simulink model "siWDqudong_FAN_MPC"  (R2024b)
settings: Solver=ode4  StartTime=0.0  StopTime=30  FixedStep=0.0005  RelTol=1e-3
undefined symbols (not defined in the file): MotorData, Q_beta_tune, Q_yaw_tune, R_alloc_tune, R_rate_tune, Road_Curvature_Map, Road_Mu_Map, Sim_Mu_Set, Sim_Vx_Set, Target_Speed_Map, W_util_tune
libraries: Solver_SF x1
(part 3 of 3)

== matlab function siWDqudong_FAN_MPC/Subsystem1/MATLAB Function ==
  data: x_curr input; T_final_opt output; Solver_Status output; x_ref input; T_ref_upper_in input size=[4 1]; Vehicle_State input; Stiffness_Input input size=[2 1]; NN_Weights input; Constraints input; dt_in input; Mu_in input; Curv_in input; Delta_f_in input; Debug_Info output size=[5 1]
function [T_final_opt, Solver_Status, Debug_Info] = Lower_Layer_MPC_Fixed(...
    x_curr, x_ref, T_ref_upper_in, Vehicle_State, Stiffness_Input, ...
    NN_Weights, Constraints, dt_in, Mu_in, Curv_in, Delta_f_in)
%#codegen
% =========================================================================
% 下层四轮LTV-MPC V6.2 dynamic W_util
%
% 直接替换原 Lower_Layer_MPC_Fixed。
% 输入/输出接口保持不变。
%
% 主要修正：
% 1) 使用可解释的无量纲物理归一化cost；
% 2) Np=25, Nc=2，Nc以后保持最后控制量；
% 3) 真正硬约束：
%       |u1-u_prev| <= dT_rate_max*dt
%       |u2-u1|     <= dT_rate_max*dt
% 4) Constraints(3) 明确定义为 Nm/s。
%    若 Constraints=[-200,800,600] 且dt=0.01，则du_max=6 Nm/step；
% 5) 不再使用8000 Nm/s的默认超大变化率去“放任抖振”；
% 6) 电机上下限使用Constraints(1/2)，同时仍限制到车辆实际±350 Nm范围；
% 7) BO/BPNN权重为无量纲乘子；搜索域与V5归一化定义同步；
% 8) fallback优先满足当前轮胎/电机安全边界；
% 9) 参考转矩只做轻度低通，避免与上层形成过重双重延迟。
% 10) 原 W_slip 重构为 W_util：按每轮动态剩余纵向能力连续归一化，无固定软阈值。
% =========================================================================

%% 0. 初始化
T_final_opt = zeros(4,1,'double');
Solver_Status = 0.0;
Debug_Info = zeros(5,1,'double');

%% 1. 输入
Veh_State = double(reshape(Vehicle_State,6,1));

Vx = max(Veh_State(1),1.0);

Fz_floor = 100.0;
Fz_fl_raw = max(Veh_State(3),Fz_floor);
Fz_fr_raw = max(Veh_State(4),Fz_floor);
Fz_rl_raw = max(Veh_State(5),Fz_floor);
Fz_rr_raw = max(Veh_State(6),Fz_floor);

dt = double(dt_in(1));
if dt <= 0
    dt = 0.01;
end

beta_in = double(x_curr(1));
r_in = double(x_curr(2));
x_ref_safe = double(reshape(x_ref,2,1));

delta_f_rad = double(Delta_f_in(1));

mu_est = min(max(double(Mu_in(1)),0.15),1.20);

kappa_abs = abs(double(Curv_in(1)));

%% 2. persistent
persistent u_prev
persistent Fz_fl_f Fz_fr_f Fz_rl_f Fz_rr_f
persistent T_ref_f
persistent logW_prev
persistent weight_initialized

if isempty(u_prev)
    u_prev = zeros(4,1);

    Fz_fl_f = Fz_fl_raw;
    Fz_fr_f = Fz_fr_raw;
    Fz_rl_f = Fz_rl_raw;
    Fz_rr_f = Fz_rr_raw;

    T_ref_f = double(reshape(T_ref_upper_in,4,1));

    logW_prev = [log10(2000.0);log10(125.0);log10(3000.0);log10(480.0);log10(1.0)];
    weight_initialized = false;
end

%% 3. Fz滤波
tau_Fz = 0.06;
alpha_Fz = dt/(tau_Fz+dt);

Fz_fl_f = Fz_fl_f + alpha_Fz*(Fz_fl_raw-Fz_fl_f);
Fz_fr_f = Fz_fr_f + alpha_Fz*(Fz_fr_raw-Fz_fr_f);
Fz_rl_f = Fz_rl_f + alpha_Fz*(Fz_rl_raw-Fz_rl_f);
Fz_rr_f = Fz_rr_f + alpha_Fz*(Fz_rr_raw-Fz_rr_f);

Fz_fl = Fz_fl_f;
Fz_fr = Fz_fr_f;
Fz_rl = Fz_rl_f;
Fz_rr = Fz_rr_f;

Fz_total = Fz_fl+Fz_fr+Fz_rl+Fz_rr;

% 硬安全边界使用raw和filtered中较保守者
Fz_fl_safe = max(min(Fz_fl_raw,Fz_fl_f),Fz_floor);
Fz_fr_safe = max(min(Fz_fr_raw,Fz_fr_f),Fz_floor);
Fz_rl_safe = max(min(Fz_rl_raw,Fz_rl_f),Fz_floor);
Fz_rr_safe = max(min(Fz_rr_raw,Fz_rr_f),Fz_floor);

%% 4. 上层参考只做轻度平滑
T_ref_raw = double(reshape(T_ref_upper_in,4,1));

tau_ref = 0.035;
alpha_ref = dt/(tau_ref+dt);

T_ref_f = T_ref_f + alpha_ref*(T_ref_raw-T_ref_f);

T_ref_upper = T_ref_f;
T_total_req = sum(T_ref_upper);

%% 5. 权重：BO训练域投影 + log变化率限制
W_in = double(reshape(NN_Weights,5,1));
W_in = max(W_in,1e-12);

logW_raw = log10(W_in);

log_lo = [0.0;0.7958800173;1.0;-3.0;-3.0];
log_hi = [4.5;3.2958800173;5.5;3.7041199827;4.0];

for ii=1:5
    logW_raw(ii)=min(max(logW_raw(ii),log_lo(ii)),log_hi(ii));
end

dlog_max = [0.08;0.08;0.10;0.10;0.10];

if ~weight_initialized
    logW_eff = logW_raw;
    weight_initialized = true;
else
    dlog = logW_raw-logW_prev;

    for ii=1:5
        dlog(ii)=min(max(dlog(ii),-dlog_max(ii)),dlog_max(ii));
    end

    logW_eff = logW_prev+dlog;
end

logW_prev = logW_eff;

W_eff = 10.^logW_eff;

Q_beta_raw  = W_eff(1);
Q_yaw_raw   = W_eff(2);
R_alloc_raw = W_eff(3);
R_rate_raw  = W_eff(4);
W_util_raw  = W_eff(5);

%% 6. 物理归一化
% Characteristic scales for dimensionless MPC cost
% beta_s : characteristic sideslip error [rad]
% r_s    : characteristic yaw-rate tracking error [rad/s]
% T_s    : characteristic single-wheel torque error [Nm]
% dT_s   : nominal one-step torque increment at 2000 Nm/s, dt=0.01 s [Nm]
% Tsum_s : four-wheel total-torque characteristic scale [Nm]
beta_s = 0.05;
r_s    = 0.10;
T_s    = 100.0;
dT_s   = 20.0;
Tsum_s = 400.0;

Q_beta = Q_beta_raw/(beta_s^2);
Q_yaw  = Q_yaw_raw /(r_s^2);

R_alloc = R_alloc_raw/(T_s^2);

R_rate_base = R_rate_raw/(dT_s^2);
R_rate_vec = R_rate_base*ones(4,1);

% q_sum is rescaled from the old 90000/320^2 so the working baseline
% effective total-demand penalty is exactly preserved after Tsum_s=400 Nm.
W_sum = 140625.0/(Tsum_s^2);

Re = 0.347;

% V6.2: dynamic remaining longitudinal tire capacity.
% No fixed 0.80/0.85 utilization threshold is used. The soft penalty grows
% continuously as mu decreases, Fz unloads, or lateral demand increases.
D_lat = Vx*Vx*kappa_abs/max(mu_est*9.81,1e-6);
gamma_mu = 1.00;  % physical friction-circle boundary, not a soft threshold
friction_factor = sqrt(max(gamma_mu^2-D_lat^2,0.0));

T_dyn_fl = Fz_fl_safe*mu_est*friction_factor*Re;
T_dyn_fr = Fz_fr_safe*mu_est*friction_factor*Re;
T_dyn_rl = Fz_rl_safe*mu_est*friction_factor*Re;
T_dyn_rr = Fz_rr_safe*mu_est*friction_factor*Re;

% Smooth denominator prevents numerical singularity without introducing a
% fixed switching threshold. J_util ~= W_util * sum((T_i/T_cap_i)^2).
T_util_eps = 5.0;
T_util_scale = sqrt([T_dyn_fl^2;T_dyn_fr^2;T_dyn_rl^2;T_dyn_rr^2] + T_util_eps^2);
W_util_vec = W_util_raw./(T_util_scale.^2);

%% 7. LTV模型
Cf = max(double(Stiffness_Input(1)),1000.0);
Cr = max(double(Stiffness_Input(2)),1000.0);

Np = 25;
Nc = 2;
nx = 2;
nu = 4;

m  = 1810.0;
Iz = 2765.0;
lf = 1.152;
lr = 1.528;
twf = 1.565;
twr = 1.565;

a11 = -(Cf+Cr)/(m*Vx);
a12 = ((lr*Cr-lf*Cf)/(m*Vx^2))-1.0;
a21 = (lr*Cr-lf*Cf)/Iz;
a22 = -(lf^2*Cf+lr^2*Cr)/(Iz*Vx);

A = eye(nx)+[a11,a12;a21,a22]*dt;

B_row2 = [ ...
    -twf/(2*Re*Iz), ...
     twf/(2*Re*Iz), ...
    -twr/(2*Re*Iz), ...
     twr/(2*Re*Iz)]*dt;

B = [zeros(1,4);B_row2];

B_delta_cont = [Cf/(m*Vx);lf*Cf/Iz];
B_delta = B_delta_cont*dt;

%% 8. 预测矩阵
Phi = zeros(nx*Np,nx);
Gamma = zeros(nx*Np,nu*Nc);
Gamma_delta = zeros(nx*Np,1);

for i=1:Np
    rows_i=(i-1)*nx+(1:nx);

    Phi(rows_i,:)=A^i;

    % steering在预测域中保持当前值
    Gd=zeros(nx,1);
    for q=0:(i-1)
        Gd=Gd+(A^q)*B_delta;
    end
    Gamma_delta(rows_i,:)=Gd;

    for j=1:min(i,Nc)
        cols_j=(j-1)*nu+(1:nu);

        if j < Nc
            term=(A^(i-j))*B;
        else
            % 第Nc个控制量保持至预测域结束
            term=zeros(nx,nu);

            for q=0:(i-Nc)
                term=term+(A^q)*B;
            end
        end

        Gamma(rows_i,cols_j)=term;
    end
end

%% 9. Cost
Q_bar = kron(eye(Np),diag([Q_beta;Q_yaw]));

H_stab = Gamma'*Q_bar*Gamma;

X_free = Phi*[beta_in;r_in]+Gamma_delta*delta_f_rad;
Y_ref = repmat(x_ref_safe,Np,1);

f_stab = (X_free-Y_ref)'*Q_bar*Gamma;

% 9.1 nominal torque reference
R_alloc_mat = diag(repmat(R_alloc*ones(nu,1),Nc,1));

H_alloc = R_alloc_mat;

U_ref_vec = repmat(T_ref_upper,Nc,1);

f_alloc = -U_ref_vec'*R_alloc_mat;

% 9.2 torque rate
D = zeros(nu*Nc,nu*Nc);

for k=1:Nc
    rows=(k-1)*nu+(1:nu);
    cols=(k-1)*nu+(1:nu);

    D(rows,cols)=eye(nu);

    if k>1
        D(rows,cols-nu)=-eye(nu);
    end
end

R_rate_diag = repmat(R_rate_vec,Nc,1);
R_w_mat = diag(R_rate_diag);

H_rate = D'*R_w_mat*D;

d0=zeros(nu*Nc,1);
d0(1:nu)=u_prev;

f_rate = -d0'*R_w_mat*D;

% 9.3 total demand soft tracking
H_sum=zeros(nu*Nc,nu*Nc);
f_sum=zeros(1,nu*Nc);

for k_step=1:Nc
    idx=(k_step-1)*nu+(1:nu);

    H_sum(idx,idx)=W_sum*ones(nu,nu);
    f_sum(idx)=-W_sum*T_total_req*ones(1,nu);
end

% 9.4 dynamic tire-utilization term
H_util = diag(repmat(W_util_vec,Nc,1));
f_util = zeros(1,nu*Nc);

% 9.5 final
H=2*(H_stab+H_alloc+H_rate+H_sum+H_util);

f=2*(f_stab+f_alloc+f_rate+f_sum+f_util)';

H=(H+H')/2+1e-6*eye(size(H));

%% 10. 动态转矩边界
Cons = double(reshape(Constraints,[],1));

% 电机物理范围
T_motor_min = -350.0;
T_motor_max =  350.0;

if numel(Cons)>=1 && isfinite(Cons(1))
    T_motor_min = max(double(Cons(1)),-350.0);
end

if numel(Cons)>=2 && isfinite(Cons(2))
    T_motor_max = min(double(Cons(2)),350.0);
end

if T_motor_min > T_motor_max
    temp = T_motor_min;
    T_motor_min = T_motor_max;
    T_motor_max = temp;
end

% T_dyn_* 已在 cost 构造前按同一动态摩擦圆计算。
% 这里仅将该物理能力作为每轮动态 box 约束；它随 mu/Fz/kappa 连续变化。

ub_base = [ ...
    min(T_dyn_fl,T_motor_max); ...
    min(T_dyn_fr,T_motor_max); ...
    min(T_dyn_rl,T_motor_max); ...
    min(T_dyn_rr,T_motor_max)];

lb_base = [ ...
    max(-T_dyn_fl,T_motor_min); ...
    max(-T_dyn_fr,T_motor_min); ...
    max(-T_dyn_rl,T_motor_min); ...
    max(-T_dyn_rr,T_motor_min)];

ub = repmat(ub_base,Nc,1);
lb = repmat(lb_base,Nc,1);

%% 11. 真正的硬件变化率约束
% 重要：
% Constraints(3) = Nm/s，不是Nm/step。
% 例如600 Nm/s，在dt=0.01时就是6 Nm/step。
dT_rate_max = 2000.0; % default Nm/s

if numel(Cons)>=3 && isfinite(Cons(3)) && Cons(3)>0
    dT_rate_max = abs(double(Cons(3)));
end

du_max = dT_rate_max*dt;

% 防止错误配置为极小/极大值
du_max = min(max(du_max,0.5),30.0);

du_vec = du_max*ones(nu*Nc,1);

A_du = [D;-D];
b_du = [du_vec+d0;du_vec-d0];

%% 12. QP
coder.extrinsic('quadprog');
coder.extrinsic('optimoptions');

options=optimoptions('quadprog', ...
    'Display','off', ...
    'Algorithm','interior-point-convex');

U0 = repmat(u_prev,Nc,1);

% 先投影到box
U0 = min(max(U0,lb),ub);

[U_mx,~,flag_mx]=quadprog( ...
    H,f, ...
    A_du,b_du, ...
    [],[], ...
    lb,ub, ...
    U0,options);

flag=-1;

if ~isempty(flag_mx)
    flag=double(flag_mx);
end

U_native=zeros(nu*Nc,1);

if ~isempty(U_mx)
    U_native=double(U_mx);
end

%% 13. 输出
if flag>0
    T_out=U_native(1:4);
    Solver_Status=1.0;
else
    % QP失败时：安全优先。
    % 先将上层参考投影到当前动态box。
    T_box = min(max(T_ref_upper,lb_base),ub_base);

    % 再尝试满足rate约束
    lower_rate = u_prev-du_max;
    upper_rate = u_prev+du_max;

    T_rate = min(max(T_box,lower_rate),upper_rate);

    % 若rate区间和安全box有交集，采用交集内结果；
    % 若没有交集（例如安全能力突然骤降），优先满足安全box。
    T_out = T_box;

    for ii=1:4
        int_lo=max(lb_base(ii),lower_rate(ii));
        int_hi=min(ub_base(ii),upper_rate(ii));

        if int_lo <= int_hi
            T_out(ii)=min(max(T_box(ii),int_lo),int_hi);
        else
            T_out(ii)=T_box(ii);
        end
    end

    Solver_Status=-1.0;
end

%% 14. 最终数值保护
for ii=1:4
    if isnan(T_out(ii)) || isinf(T_out(ii))
        T_out(ii)=0.0;
    elseif abs(T_out(ii))<2.0
        T_out(ii)=0.0;
    end

    T_out(ii)=min(max(T_out(ii),lb_base(ii)),ub_base(ii));
end

u_prev=T_out;
T_final_opt(:)=T_out;

%% 15. Debug
% 1 effective Q_beta
% 2 effective R_alloc
% 3 du_max [Nm/step]
% 4 D_lat
% 5 solver status
Debug_Info(:)=[Q_beta;R_alloc;du_max;D_lat;Solver_Status];

end
